simulink model "SFpolytopic"  (R2018b)
settings: Solver=VariableStepAuto  StartTime=0.0  StopTime=10.0  RelTol=1e-3
undefined symbols (not defined in the file or in its folder): K1, K2, K3, K4, rho1max, rho1min, rho2max, rho2min
settings Model: Creator=senameo  LastModifiedBy=senameo

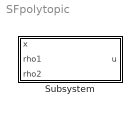
== system SFpolytopic ==
  Subsystem : Subsystem

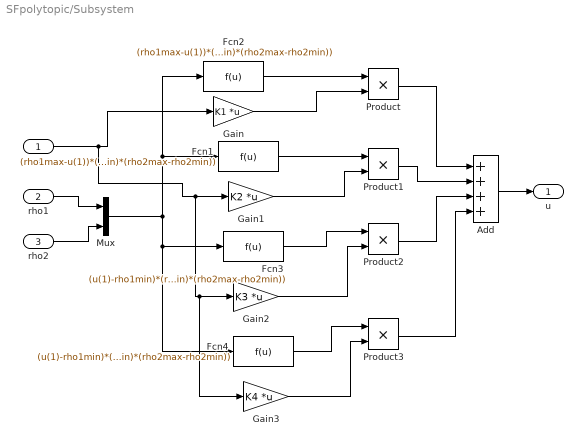
== system SFpolytopic/Subsystem ==
  x : Inport
  rho1 : Inport  Port=2
  rho2 : Inport  Port=3
  Add : Sum  Inputs=++++
  Fcn1 : Fcn  Expr=(rho1max-u(1))*(u(2)-rho2min)/((rho1max-rho1min)*(rho2max-rho2min))
  Fcn2 : Fcn  Expr=(rho1max-u(1))*(rho2max-u(2))/((rho1max-rho1min)*(rho2max-rho2min))
  Fcn3 : Fcn  Expr=(u(1)-rho1min)*(rho2max-u(2))/((rho1max-rho1min)*(rho2max-rho2min))
  Fcn4 : Fcn  Expr=(u(1)-rho1min)*(u(2)-rho2min)/((rho1max-rho1min)*(rho2max-rho2min))
  Gain : Gain  Gain=K1  Multiplication=Matrix(K*u)
  Gain1 : Gain  Gain=K2  Multiplication=Matrix(K*u)
  Gain2 : Gain  Gain=K3  Multiplication=Matrix(K*u)
  Gain3 : Gain  Gain=K4  Multiplication=Matrix(K*u)
  Mux : Mux  Inputs=2
  Product{,1..3} (4 alike) : Product
  "u " : Outport
  wires:
  Fcn2/1 -> Product/1
  Gain/1 -> Product/2
  Product/1 -> Add/1
  Product1/1 -> Add/2
  Gain1/1 -> Product1/2
  Fcn1/1 -> Product1/1
  Add/1 -> "u "/1
  rho1/1 -> Mux/1
  rho2/1 -> Mux/2
  Mux/1 -> Fcn1/1, Fcn2/1, Fcn4/1, Fcn3/1
  Product2/1 -> Add/3
  Product3/1 -> Add/4
  Fcn4/1 -> Product3/1
  Gain3/1 -> Product3/2
  Fcn3/1 -> Product2/1
  Gain2/1 -> Product2/2
  x/1 -> Gain3/1, Gain2/1, Gain1/1, Gain/1
